simulink model "Robot_AdpG"  (Simulink 8.0)
settings: Solver=ode45  StartTime=0.0  StopTime=simtime  RelTol=1e-3
values from neighbouring files (symbols this model uses):
  Gamma = 200 * Gamma0_G    [robot_master.m]
  Lambda = 20 * eye(2, 2)    [robot_master.m]
settings Model: Creator=Dan  LastModifiedBy=Dan
settings DataIOCC: SignalLoggingSaveFormat=ModelDataLogs
settings DebuggingCC: FcnCallInpInsideContextMsg=UseLocalSettings
settings GRTTargetCC: CombineOutputUpdateFcns=off  GRTInterface=on

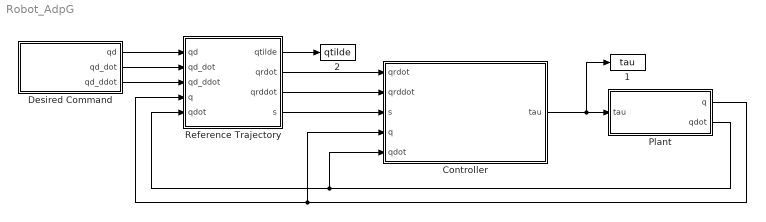
== system Robot_AdpG ==
  1 : ToWorkspace  VariableName=tau  SampleTime=-1
  2 : ToWorkspace  VariableName=qtilde  SampleTime=-1
  Controller : Subsystem
  Desired Command : Subsystem
  Plant : Subsystem
  Reference Trajectory : Subsystem
  wires:
  Plant/2(qdot) -> Reference Trajectory/5(qdot), Controller/5(qdot)
  Plant/1(q) -> Reference Trajectory/4(q), Controller/4(q)
  Reference Trajectory/2(qrdot) -> Controller/1(qrdot)
  Reference Trajectory/3(qrddot) -> Controller/2(qrddot)
  Reference Trajectory/1(qtilde) -> 2/1
  Reference Trajectory/4(s) -> Controller/3(s)
  Controller/1(tau) -> 1/1, Plant/1(tau)
  Desired Command/1(qd) -> Reference Trajectory/1(qd)
  Desired Command/2(qd_dot) -> Reference Trajectory/2(qd_dot)
  Desired Command/3(qd_ddot) -> Reference Trajectory/3(qd_ddot)

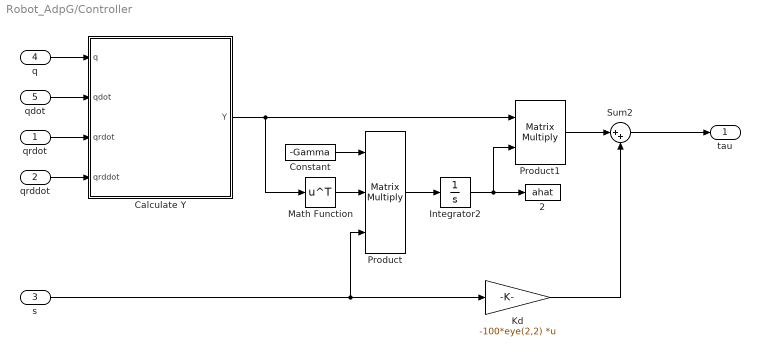
== system Robot_AdpG/Controller ==
  qrdot : Inport
  qrddot : Inport  Port=2
  s : Inport  Port=3
  q : Inport  Port=4
  qdot : Inport  Port=5
  2 : ToWorkspace  VariableName=ahat  SampleTime=-1
  Calculate Y : MATLAB Function  TreatAsAtomicUnit=on
  Constant : Constant  Value=-Gamma
  Integrator2 : Integrator  InitialCondition=[0;0;0;0;0;0;0];
  Kd : Gain  Gain=-100*eye(2,2)  Multiplication=Matrix(K*u)
  Math Function : Math  Operator=transpose  SaturateOnIntegerOverflow=on
  Product : Product  Inputs=3  Multiplication=Matrix(*)  RndMeth=Zero
  Product1 : Product  Multiplication=Matrix(*)  RndMeth=Zero
  Sum2 : Sum  Inputs=|++
  tau : Outport
  wires:
  Calculate Y/1(Y) -> Math Function/1, Product1/1
  Constant/1 -> Product/1
  Math Function/1 -> Product/2
  s/1 -> Kd/1, Product/3
  Product/1 -> Integrator2/1
  Integrator2/1 -> Product1/2, 2/1
  Product1/1 -> Sum2/1
  Kd/1 -> Sum2/2
  Sum2/1 -> tau/1
  q/1 -> Calculate Y/1(q)
  qdot/1 -> Calculate Y/2(qdot)
  qrdot/1 -> Calculate Y/3(qrdot)
  qrddot/1 -> Calculate Y/4(qrddot)

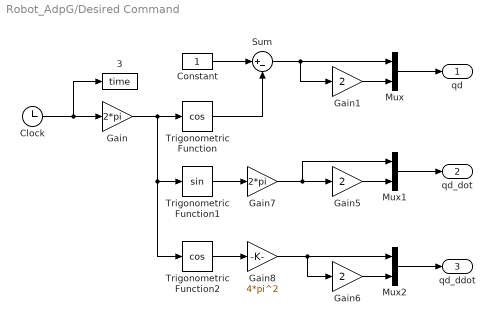
== system Robot_AdpG/Desired Command ==
  3 : ToWorkspace  VariableName=time  SampleTime=-1
  Clock : Clock
  Constant : Constant
  Gain : Gain  Gain=2*pi
  Gain1 : Gain  Gain=2
  Gain5 : Gain  Gain=2
  Gain6 : Gain  Gain=2
  Gain7 : Gain  Gain=2*pi
  Gain8 : Gain  Gain=4*pi^2
  Mux : Mux  Inputs=2
  Mux1 : Mux  Inputs=2
  Mux2 : Mux  Inputs=2
  Sum : Sum  Inputs=|+-
  Trigonometric Function : Trigonometry  Operator=cos
  Trigonometric Function1 : Trigonometry
  Trigonometric Function2 : Trigonometry  Operator=cos
  qd : Outport
  qd_dot : Outport  Port=2
  qd_ddot : Outport  Port=3
  wires:
  Clock/1 -> Gain/1, 3/1
  Gain/1 -> Trigonometric Function/1, Trigonometric Function1/1, Trigonometric Function2/1
  Constant/1 -> Sum/1
  Trigonometric Function/1 -> Sum/2
  Sum/1 -> Mux/1, Gain1/1
  Gain1/1 -> Mux/2
  Trigonometric Function1/1 -> Gain7/1
  Gain7/1 -> Mux1/1, Gain5/1
  Trigonometric Function2/1 -> Gain8/1
  Gain8/1 -> Gain6/1, Mux2/1
  Mux/1 -> qd/1
  Gain5/1 -> Mux1/2
  Gain6/1 -> Mux2/2
  Mux1/1 -> qd_dot/1
  Mux2/1 -> qd_ddot/1

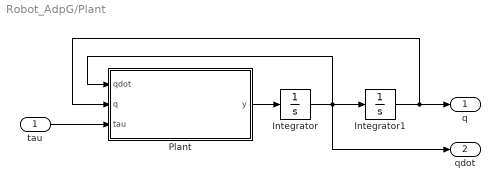
== system Robot_AdpG/Plant ==
  tau : Inport
  Integrator : Integrator  InitialCondition=[0;0];
  Integrator1 : Integrator  InitialCondition=[0;0];
  Plant : MATLAB Function  TreatAsAtomicUnit=on
  q : Outport
  qdot : Outport  Port=2
  wires:
  Plant/1(y) -> Integrator/1
  Integrator/1 -> qdot/1, Integrator1/1, Plant/1(qdot)
  Integrator1/1 -> q/1, Plant/2(q)
  tau/1 -> Plant/3(tau)

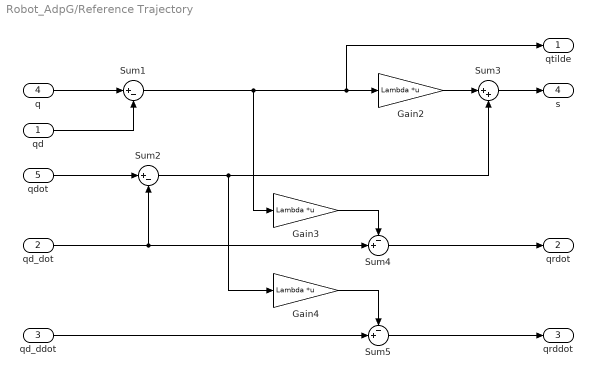
== system Robot_AdpG/Reference Trajectory ==
  qd : Inport
  qd_dot : Inport  Port=2
  qd_ddot : Inport  Port=3
  q : Inport  Port=4
  qdot : Inport  Port=5
  Gain2 : Gain  Gain=Lambda  Multiplication=Matrix(K*u)
  Gain3 : Gain  Gain=Lambda  Multiplication=Matrix(K*u)
  Gain4 : Gain  Gain=Lambda  Multiplication=Matrix(K*u)
  Sum1 : Sum  Inputs=|+-
  Sum2 : Sum  Inputs=|+-
  Sum3 : Sum  Inputs=|++
  Sum4 : Sum  Inputs=-+|
  Sum5 : Sum  Inputs=-+|
  qtilde : Outport
  qrdot : Outport  Port=2
  qrddot : Outport  Port=3
  s : Outport  Port=4
  wires:
  qd/1 -> Sum1/2
  qd_dot/1 -> Sum2/2, Sum4/2
  q/1 -> Sum1/1
  Sum1/1 -> Gain3/1, qtilde/1, Gain2/1
  qdot/1 -> Sum2/1
  Sum2/1 -> Sum3/2, Gain4/1
  Gain2/1 -> Sum3/1
  Sum3/1 -> s/1
  Sum4/1 -> qrdot/1
  Sum5/1 -> qrddot/1
  Gain3/1 -> Sum4/1
  Gain4/1 -> Sum5/1
  qd_ddot/1 -> Sum5/2

== matlab function Controller/Calculate Y ==
  data: q input double; Y output double; qdot input double; qrdot input double; qrddot input double
%%%%%%%%%%%%%%%%%%%%%%%%%%%%%%%%%%%%%%%%%%%%%%%%%%%%%%%%%%%%%%%%%%%%%%%%%%%
% Daniel Wiese
% 2.152
% Robot Manipulator
%--------------------------------------------------------------------------
% Robot
%%%%%%%%%%%%%%%%%%%%%%%%%%%%%%%%%%%%%%%%%%%%%%%%%%%%%%%%%%%%%%%%%%%%%%%%%%%
function Y=fcn(q,qdot,qrdot,qrddot)
%#codegen
%Preallocate output
Y=zeros(2,7);
%Take apart the input
q1=q(1);
q2=q(2);
qdot1=qdot(1);
qdot2=qdot(2);
qrdot1=qrdot(1);
qrdot2=qrdot(2);
qrddot1=qrddot(1);
qrddot2=qrddot(2);
%Calculate the first row of Y
Y(1,1)=qrddot1;
Y(1,2)=qrddot2;
Y(1,3)=(2*qrddot1+qrddot2)*cos(q2)-(qdot2*qrdot1+qdot1*qrdot2+qdot2*qrdot2)*sin(q2);
Y(1,4)=(2*qrddot1+qrddot2)*sin(q2)+(qdot2*qrdot1+qdot1*qrdot2+qdot2*qrdot2)*cos(q2);
Y(1,5)=cos(q1);
Y(1,6)=cos(q1+q2);
Y(1,7)=-sin(q1+q2);
%Calculate the second row of Y
Y(2,1)=0;
Y(2,2)=qrddot1+qrddot2;
Y(2,3)=qrddot1*cos(q2)+qdot1*qrdot1*sin(q2);
Y(2,4)=qrddot1*sin(q2)-qdot1*qrdot1*cos(q2);
Y(2,5)=0;
Y(2,6)=cos(q1+q2);
Y(2,7)=-sin(q1+q2);

== matlab function Plant/Plant ==
  data: qdot input double; q input double; y output double; tau input double
%%%%%%%%%%%%%%%%%%%%%%%%%%%%%%%%%%%%%%%%%%%%%%%%%%%%%%%%%%%%%%%%%%%%%%%%%%%
% Daniel Wiese
% 2.152
% Robot Manipulator
%--------------------------------------------------------------------------
% Robot manipulator. See Slotine, Li page 396 for the equations and all of
% the parameter values used.
%%%%%%%%%%%%%%%%%%%%%%%%%%%%%%%%%%%%%%%%%%%%%%%%%%%%%%%%%%%%%%%%%%%%%%%%%%%
function y = fcn(qdot,q,tau)
%#codegen
%Take apart the input
q1=q(1);
q2=q(2);
qdot1=qdot(1);
qdot2=qdot(2);
g=9.81;
%Plant parameters
M1=1;
L1=1;
Me=2;
de=30*pi/180;
I1=0.12;
Lc1=0.5;
Ie=0.25;
Lce=0.6;
%Define the 'a' parameters
a1=I1+M1*Lc1^2+Ie+Me*Lc1^2+Me*L1^2;
a2=Ie+Me*Lce^2;
a3=Me*L1*Lce*cos(de);
a4=Me*L1*Lce*sin(de);
%Components of the matrix H
H11=a1+2*a3*cos(q2)+2*a4*sin(q2);
H12=a2+a3*cos(q2)+a4*sin(q2);
H21=H12;
H22=a2;
h=a3*sin(q2)-a4*cos(q2);
%The gravity matrix G
G=[(M1*Lc1+Me*L1)*g*cos(q1)+((Me*Lce*g)/cos(de))*cos(q1+q2+de);
    ((Me*Lce*g)/cos(de))*cos(q1+q2+de)];
%Assemble H and C
H=[H11 H12; H21 H22];
C=[-h*qdot2 -h*(qdot1+qdot2); h*qdot1 0];
%Calculate the plant output y=q_ddot
y = -inv(H)*C*qdot+inv(H)*tau+inv(H)*G;
